simulink model "Step_input"  (R2020b)
settings: Solver=VariableStepAuto  StartTime=0.0  StopTime=10.0  RelTol=1e-3
values from neighbouring files (symbols this model uses):
  c1 = 100    [parameters.m]
  c2 = 1000    [parameters.m]
  k1 = 1e4    (= 10000)    [parameters.m]
  k2 = 1e5    (= 100000)    [parameters.m]
  m1 = 10    [parameters.m]
  m2 = 100    [parameters.m]
settings Model: Creator=bhuva  LastModifiedBy=bhuva

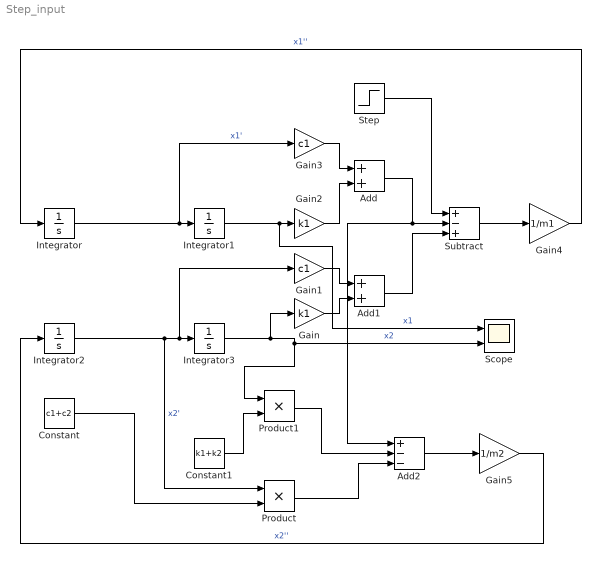
== system Step_input ==
  Add : Sum
  Add1 : Sum
  Add2 : Sum  Inputs=+--
  Constant : Constant  Value=c1+c2
  Constant1 : Constant  Value=k1+k2
  Gain : Gain  Gain=k1
  Gain1 : Gain  Gain=c1
  Gain2 : Gain  Gain=k1
  Gain3 : Gain  Gain=c1
  Gain4 : Gain  Gain=1/m1
  Gain5 : Gain  Gain=1/m2
  Integrator{,1..3} (4 alike) : Integrator
  Product : Product
  Product1 : Product
  Scope : Scope  NumInputPorts=2
  Step : Step  After=5  SampleTime=0
  Subtract : Sum  Inputs=+-+
  wires:
  Integrator/1 -> Gain3/1, Integrator1/1  "x1'"
  Integrator1/1 -> Scope/1, Gain2/1  "x1"
  Gain4/1 -> Integrator/1  "x1''"
  Integrator2/1 -> Gain1/1, Integrator3/1, Product/1  "x2'"
  Gain5/1 -> Integrator2/1  "x2''"
  Integrator3/1 -> Product1/1, Scope/2, Gain/1  "x2"
  Constant/1 -> Product/2
  Constant1/1 -> Product1/2
  Gain3/1 -> Add/1
  Gain2/1 -> Add/2
  Gain1/1 -> Add1/1
  Gain/1 -> Add1/2
  Step/1 -> Subtract/1
  Add/1 -> Add2/1, Subtract/2
  Add1/1 -> Subtract/3
  Subtract/1 -> Gain4/1
  Product1/1 -> Add2/2
  Product/1 -> Add2/3
  Add2/1 -> Gain5/1
